simulink model "threetank_FDF"  (Simulink 9.0)
settings: Solver=ode45  StartTime=0.0  StopTime=2000  RelTol=1e-3  EnableMultiTasking=on
values from neighbouring files (symbols this model uses):
  A = [eval(a11),eval(a12),eval(a13);eval(a21),eval(a22),eval(a23);eval(a31),eval(a32),eval(a33)]    [Threetank.m]
  B = [eval(b11),eval(b12);eval(b21),eval(b22);eval(b31),eval(b32)]    [Threetank.m]
  C = eye(3)    [Threetank.m]    (also in data429.m = chol(sigma_m); datageneratev51.m = chol(sigma_m))
  D = zeros(3,2)    [Threetank.m]
  Ed = zeros(3,2)    [Threetank.m]
  Ef = [zeros(3,3),B]    [Threetank.m]
  Fd = [1,0;0,1;0,0]    [Threetank.m]
  Ff = [eye(3),zeros(3,2)]    [Threetank.m]
  L_FDF = place(A',C',[1.5*eig(A)])'    [Threetank.m]
  sys = ss(A,B,C,D)    [Threetank.m]    (also in collectdata.m = [])
libraries: simulink x2
settings Model: SuppressorTable=22 serialization::archive 11 0 6 0 0 0 0 0  Creator=AKS USER  LastModifiedBy=zhongcheng
settings DataIOCC: LimitDataPoints=on  SignalLoggingSaveFormat=ModelDataLogs
settings OptimizationCC: InitFltsAndDblsToZero=on
settings DebuggingCC: SaveWithParameterizedLinksMsg=none  SignalResolutionControl=TryResolveAllWithWarning  SolverPrmCheckMsg=warning  FcnCallInpInsideContextMsg=warning  StrictBusMsg=Warning
settings GRTTargetCC: TargetFcnLib=ansi_tfl_tmw.mat  CombineOutputUpdateFcns=off  GRTInterface=on

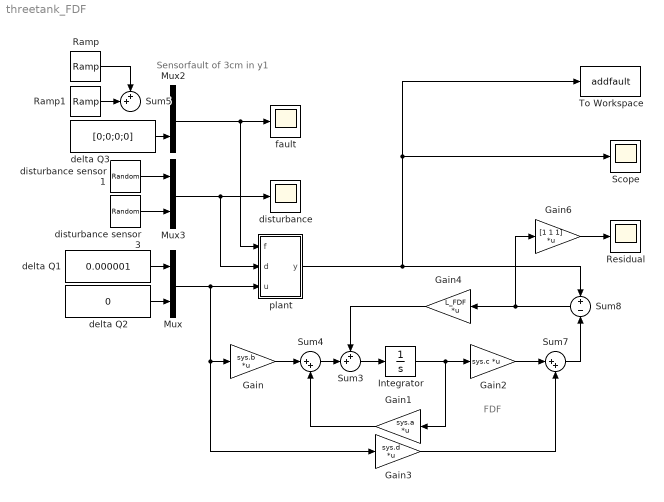
== system threetank_FDF ==
  note: FDF
  note: Sensorfault of 3cm in y1
  Gain : Gain  Gain=sys.b  Multiplication=Matrix(K*u)
  Gain1 : Gain  Gain=sys.a  Multiplication=Matrix(K*u)
  Gain2 : Gain  Gain=sys.c  Multiplication=Matrix(K*u)
  Gain3 : Gain  Gain=sys.d  Multiplication=Matrix(K*u)
  Gain4 : Gain  Gain=L_FDF  Multiplication=Matrix(K*u)
  Gain6 : Gain  Gain=[1 1 1]  Multiplication=Matrix(K*u)
  Integrator : Integrator
  Mux : Mux  Inputs=2
  Mux2 : Mux  Inputs=2
  Mux3 : Mux  Inputs=2
  Ramp : simulink/Sources/Ramp  slope=0.001  start=50  X0=0
  Ramp1 : simulink/Sources/Ramp  slope=-0.001  start=80  X0=0
  Residual : Scope
  Scope : Scope
  Sum3 : Sum  Inputs=++|
  Sum4 : Sum  Inputs=|++
  Sum5 : Sum  Inputs=++|
  Sum7 : Sum  Inputs=|++
  Sum8 : Sum  Inputs=+-
  To Workspace : ToWorkspace  VariableName=addfault  SampleTime=0.5
  delta Q1 : Constant  Value=0.000001
  delta Q2 : Constant  Value=0
  delta Q3 : Constant  Value=[0;0;0;0]
  disturbance : Scope
  disturbance sensor 1 : UniformRandomNumber  Minimum=-0.000001  Maximum=0.000001  Seed=73354757854  SampleTime=0.03
  disturbance sensor 3 : UniformRandomNumber  Minimum=-0.000001  Maximum=0.000001  Seed=632478  SampleTime=0.03
  fault : Scope
  plant : Subsystem
  wires:
  delta Q2/1 -> Mux/2
  delta Q1/1 -> Mux/1
  Ramp/1 -> Sum5/1
  Ramp1/1 -> Sum5/2
  Mux/1 -> Gain/1, Gain3/1, plant/3(u)
  Sum3/1 -> Integrator/1
  Gain/1 -> Sum4/1
  Sum4/1 -> Sum3/2
  Integrator/1 -> Gain1/1, Gain2/1
  Gain1/1 -> Sum4/2
  Gain3/1 -> Sum7/2
  Gain2/1 -> Sum7/1
  Sum7/1 -> Sum8/2
  Sum8/1 -> Gain4/1, Gain6/1
  Gain4/1 -> Sum3/1
  Gain6/1 -> Residual/1
  Mux2/1 -> plant/1(f), fault/1
  delta Q3/1 -> Mux2/2
  Mux3/1 -> plant/2(d), disturbance/1
  disturbance sensor 1/1 -> Mux3/1
  disturbance sensor 3/1 -> Mux3/2
  plant/1(y) -> To Workspace/1, Scope/1, Sum8/1

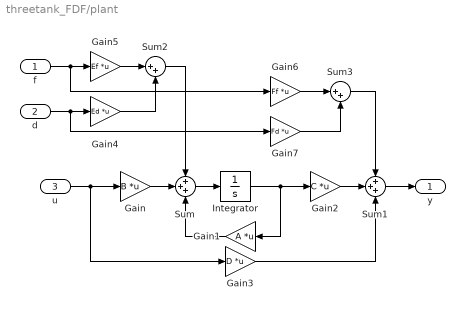
== system threetank_FDF/plant ==
  f : Inport
  d : Inport  Port=2
  u : Inport  Port=3
  Gain : Gain  Gain=B  Multiplication=Matrix(K*u)
  Gain1 : Gain  Gain=A  Multiplication=Matrix(K*u)
  Gain2 : Gain  Gain=C  Multiplication=Matrix(K*u)
  Gain3 : Gain  Gain=D  Multiplication=Matrix(K*u)
  Gain4 : Gain  Gain=Ed  Multiplication=Matrix(K*u)
  Gain5 : Gain  Gain=Ef  Multiplication=Matrix(K*u)
  Gain6 : Gain  Gain=Ff  Multiplication=Matrix(K*u)
  Gain7 : Gain  Gain=Fd  Multiplication=Matrix(K*u)
  Integrator : Integrator
  Sum : Sum  Inputs=+++
  Sum1 : Sum  Inputs=+++
  Sum2 : Sum  Inputs=|++
  Sum3 : Sum  Inputs=|++
  y : Outport
  wires:
  Sum/1 -> Integrator/1
  Integrator/1 -> Gain2/1, Gain1/1
  u/1 -> Gain/1, Gain3/1
  Gain3/1 -> Sum1/3
  Gain2/1 -> Sum1/2
  Gain/1 -> Sum/2
  Gain1/1 -> Sum/3
  Sum2/1 -> Sum/1
  Sum3/1 -> Sum1/1
  Gain4/1 -> Sum2/2
  d/1 -> Gain4/1, Gain7/1
  Gain5/1 -> Sum2/1
  f/1 -> Gain5/1, Gain6/1
  Gain6/1 -> Sum3/1
  Gain7/1 -> Sum3/2
  Sum1/1 -> y/1
